simulink model "Lab5"  (R2018a)
settings: Solver=FixedStepDiscrete  StartTime=0.0  StopTime=10  FixedStep=0.1  RelTol=1e-3  EnableMultiTasking=on
settings Model: Creator=Vadson  LastModifiedBy=Carapinha
settings SolverCC: AutoInsertRateTranBlk=on
settings DataIOCC: LimitDataPoints=on
settings OptimizationCC: LifeSpan=inf
settings DebuggingCC: AllowSymbolicDim=off  SFUnexpectedBacktrackingDiag=warning  SFNoUnconditionalDefaultTransitionDiag=warning  SFExecutionAtInitializationDiag=none
settings CodeAppCC: StateflowObjectComments=on
settings GRTTargetCC: TargetLangStandard=C89/C90 (ANSI)  GeneratePreprocessorConditionals=Disable all
settings ConfigComp: CovMetricSettings=dw  CovHtmlReporting=on  CovSaveCumulativeToWorkspaceVar=on  CovSaveSingleToWorkspaceVar=on  CovShowResultsExplorer=off  CovExternalEMLEnable=off  CovSFcnEnable=off

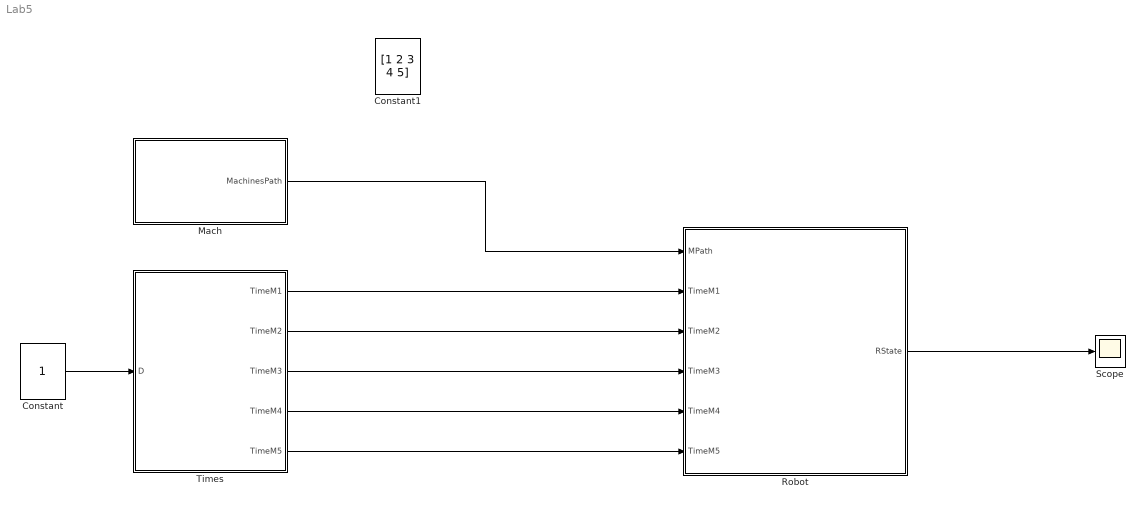
== system Lab5 ==
  Constant : Constant
  Constant1 : Constant  Value=[1 2 3 4 5]
  Mach : MATLAB Function  TreatAsAtomicUnit=on
  Robot : Stateflow chart  TreatAsAtomicUnit=on
  Scope : Scope
  Times : MATLAB Function  TreatAsAtomicUnit=on
  wires:
  Constant/1 -> Times/1(D)
  Times/5(TimeM5) -> Robot/6(TimeM5)
  Times/4(TimeM4) -> Robot/5(TimeM4)
  Times/3(TimeM3) -> Robot/4(TimeM3)
  Times/2(TimeM2) -> Robot/3(TimeM2)
  Times/1(TimeM1) -> Robot/2(TimeM1)
  Robot/1(RState) -> Scope/1
  Mach/1(MachinesPath) -> Robot/1(MPath)

== matlab function Lab5/Mach ==
  data: MachinesPath output
function MachinesPath  = Path()
j = 0;
NrProcesses = 5;
MachinesPath = zeros(1,NrProcesses);
for k=1:NrProcesses
    MachinesPath(1,k) = randi(5,1);
end

for i=1:NrProcesses-1
    if(MachinesPath(1,i) == MachinesPath(1,i+1))
        while j == 0
            A = randi(5,1);
            if(A ~= MachinesPath(1,i+1))
                if(i > 1)
                    if(A ~= MachinesPath(1,i-1))
                        MachinesPath(1,i) = A;
                        j = 1;
                    end
                else
                    p = 2;
                    if(A ~= MachinesPath(1,p-1))
                        MachinesPath(1,i) = A;
                        j = 1;
                    end
                end
            end
        end
        j = 0;
    end
end

== stateflow chart Lab5/Robot ==
  state State6
    IBufferM1 = 0;
    IBufferM2 = 0;
    IBufferM3 = 0;
    IBufferM4 = 0;
    IBufferM5 = 0;
  state State5
    RState = MPath(5);
    IBufferM5 = 1;
    OBufferM5 = 0;
    Occupied = 1;
  state State1
    RState = MPath(1);
    IBufferM1 = 1;
    OBufferM1 = 0;
    Occupied = 1;
  state idle
    if(i >= 5)
    i = 1;
    else
    i = i+1;
    end
  state State4
    RState = MPath(4);
    IBufferM4 = 1;
    OBufferM4 = 0;
    Occupied = 1;
  state State2
    RState = MPath(2);
    IBufferM2 = 1;
    OBufferM2 = 0;
    Occupied = 1;
  state State3
    RState = MPath(3);
    IBufferM3 = 1;
    OBufferM3 = 0;
    Occupied = 1;
  (default) -> State6
  State6 -> idle : {i = 0}
  State1 -> idle : [after(TimeM1, sec)]{Occupied = 0;}
  State5 -> idle : [after(TimeM5, sec)]{Occupied = 0;}
  idle -> State1 [order 5] : [MPath(i) == 1 && IBufferM1 == 0 && Occupied == 0]
  idle -> State5 [order 2] : [MPath(i) == 5  && IBufferM5 == 0 && Occupied == 0]
  idle -> State2 [order 4] : [MPath(i) == 2  && IBufferM2 == 0 && Occupied == 0]
  idle -> State4 [order 3] : [MPath(i) == 4 && IBufferM4 == 0 && Occupied == 0]
  State2 -> idle : [after(TimeM2, sec)]{Occupied = 0;}
  idle -> State3 [order 1] : [MPath(i) == 3 && IBufferM3 == 0 && Occupied == 0]
  State3 -> idle : [after(TimeM3, sec)]{Occupied = 0;}
  State4 -> idle : [after(TimeM4, sec)]{Occupied = 0;}
  data: RState output; MPath input; TimeM1 input; TimeM2 input; TimeM3 input; TimeM4 input; TimeM5 input; OBufferM5 local; IBufferM5 local; IBufferM1 local; IBufferM4 local; OBufferM1 local; IBufferM2 local; OBufferM3 local; OBufferM2 local; OBufferM4 local; IBufferM3 local; i local double; Occupied local

== matlab function Lab5/Times ==
  data: TimeM1 output; TimeM2 output; D input; TimeM3 output; TimeM4 output; TimeM5 output
function [TimeM1, TimeM2, TimeM3, TimeM4, TimeM5] = Times(D)
 
Upper = D+0.1*D;
Lower = D-0.1*D;
Range = Upper-Lower;

TimeM1 = Range*rand(1,1)+Lower;
TimeM2 = Range*rand(1,1)+Lower;
TimeM3 = Range*rand(1,1)+Lower;
TimeM4 = Range*rand(1,1)+Lower;
TimeM5 = Range*rand(1,1)+Lower;
